simulink model "controllermodel"  (R2024b)
settings: Solver=VariableStepAuto  StartTime=0.0  StopTime=10.0  RelTol=1e-3
settings Model: Creator=isaac  LastModifiedBy=isaac

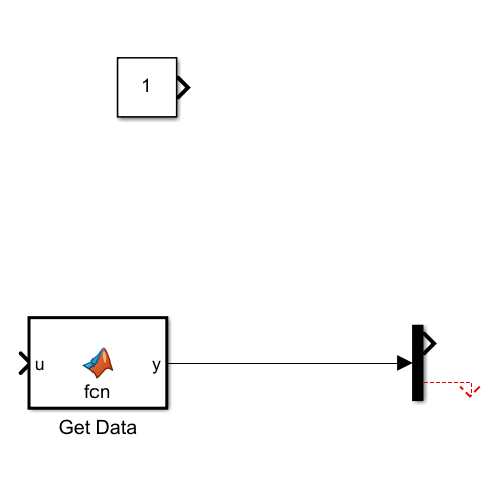
[thumbnail: Simulink's stored preview of the top-level diagram]
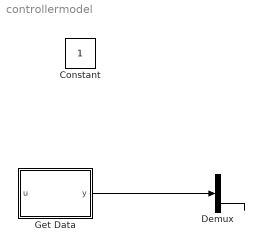
== system controllermodel ==
  Constant : Constant
  Demux : Demux  Outputs=2
  Get Data : MATLAB Function  TreatAsAtomicUnit=on
  wires:
  Get Data/1(y) -> Demux/1
  Demux/2 -> ?

== matlab function controllermodel/Get Data ==
  data: u input; y output
function y = fcn(u)
    device = serialport("COM3",9600);
    write(device,u,"uint8");
    data = read(device,5,"uint8");

y = data;
